simulink model "robot_controller"  (Simulink 8.9)
settings: Solver=ode45  StartTime=0.0  StopTime=t_final  RelTol=1e-3  EnableMultiTasking=on
values from neighbouring files (symbols this model uses):
  psi0 = 0    [CT_setup.m]    (also in plot_two_kanayama.m)
  vx_disturb = 0    [CT_setup.m]    (also in plot_two_kanayama.m)
  vy_disturb = 0    [CT_setup.m]    (also in plot_two_kanayama.m)
  w_max = 0.25    [CT_setup.m]    (also in plot_two_kanayama.m)
  w_min = -w_max    (= -0.25)    [CT_setup.m]    (also in plot_two_kanayama.m)
  x0 = 0    [CT_setup.m]    (also in plot_two_kanayama.m)
  y0 = 0    [CT_setup.m]    (also in plot_two_kanayama.m)
undefined symbols (not defined in the file or in its folder): UAV_Dynamics, UAV_with_lowlevelcontrol
libraries: simulink x1
settings Model: Creator=user  LastModifiedBy=edward
settings OptimizationCC: ExpressionDepthLimit=2147483647  InitFltsAndDblsToZero=on
settings DebuggingCC: SolverPrmCheckMsg=warning  StrictBusMsg=Warning
settings GRTTargetCC: GeneratePreprocessorConditionals=Use local settings

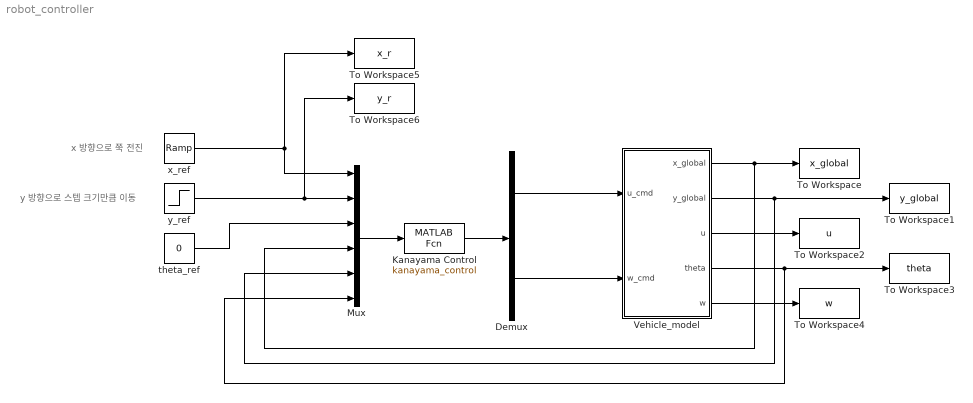
== system robot_controller ==
  note: y 방향으로 스텝 크기만큼 이동
  note: x 방향으로 쭉 전진
  Demux : Demux  Outputs=2
  Kanayama Control : MATLABFcn  MATLABFcn=kanayama_control
  Mux : Mux  Inputs=6
  To Workspace : ToWorkspace  VariableName=x_global  SampleTime=-1
  To Workspace1 : ToWorkspace  VariableName=y_global  SampleTime=-1
  To Workspace2 : ToWorkspace  VariableName=u  SampleTime=-1
  To Workspace3 : ToWorkspace  VariableName=theta  SampleTime=-1
  To Workspace4 : ToWorkspace  VariableName=w  SampleTime=-1
  To Workspace5 : ToWorkspace  VariableName=x_r  SampleTime=-1
  To Workspace6 : ToWorkspace  VariableName=y_r  SampleTime=-1
  Vehicle_model : Subsystem  AncestorBlock=UAV_Dynamics/UAV_with_lowlevelcontrol
  theta_ref : Constant  Value=0
  x_ref : simulink/Sources/Ramp  slope=1  start=0  X0=0
  y_ref : Step  Time=5  SampleTime=0
  wires:
  Vehicle_model/1(x_global) -> To Workspace/1, Mux/4
  Vehicle_model/2(y_global) -> To Workspace1/1, Mux/5
  Vehicle_model/3(u) -> To Workspace2/1
  Vehicle_model/4(theta) -> To Workspace3/1, Mux/6
  Vehicle_model/5(w) -> To Workspace4/1
  x_ref/1 -> Mux/1, To Workspace5/1
  y_ref/1 -> Mux/2, To Workspace6/1
  theta_ref/1 -> Mux/3
  Mux/1 -> Kanayama Control/1
  Kanayama Control/1 -> Demux/1
  Demux/1 -> Vehicle_model/1(u_cmd)
  Demux/2 -> Vehicle_model/2(w_cmd)

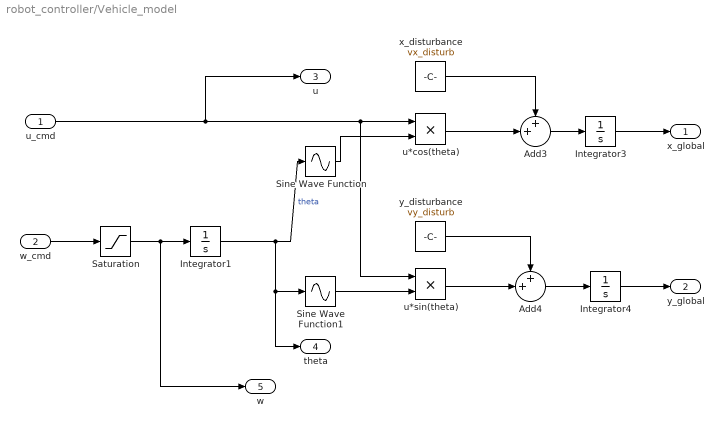
== system robot_controller/Vehicle_model ==
  u_cmd : Inport
  w_cmd : Inport  Port=2
  Add3 : Sum  Inputs=++|
  Add4 : Sum  Inputs=++|
  Integrator1 : Integrator  InitialCondition=psi0
  Integrator3 : Integrator  InitialCondition=x0
  Integrator4 : Integrator  InitialCondition=y0
  Saturation : Saturate  UpperLimit=w_max  LowerLimit=w_min
  Sine Wave Function : Sin  TimeSource=Use external signal  Phase=pi/2  SampleTime=0
  Sine Wave Function1 : Sin  TimeSource=Use external signal  SampleTime=0
  u*cos(theta) : Product  RndMeth=Zero
  u*sin(theta) : Product  RndMeth=Zero
  x_disturbance : Constant  Value=vx_disturb
  y_disturbance : Constant  Value=vy_disturb
  x_global : Outport
  y_global : Outport  Port=2
  u : Outport  Port=3
  theta : Outport  Port=4
  w : Outport  Port=5
  wires:
  Add4/1 -> Integrator4/1
  u*sin(theta)/1 -> Add4/2
  y_disturbance/1 -> Add4/1
  Add3/1 -> Integrator3/1
  u*cos(theta)/1 -> Add3/2
  x_disturbance/1 -> Add3/1
  Integrator4/1 -> y_global/1
  Integrator3/1 -> x_global/1
  Saturation/1 -> w/1, Integrator1/1
  Integrator1/1 -> Sine Wave Function/1, Sine Wave Function1/1, theta/1  "theta"
  Sine Wave Function/1 -> u*cos(theta)/2
  Sine Wave Function1/1 -> u*sin(theta)/2
  u_cmd/1 -> u*cos(theta)/1, u*sin(theta)/1, u/1
  w_cmd/1 -> Saturation/1
